simulink model "simula_RST_LPV"  (R2017a)
settings: Solver=VariableStepAuto  StartTime=0.0  StopTime=tsim  RelTol=1e-3
values from neighbouring files (symbols this model uses):
  Asim = double(A_LPV)    [Principal_LPV_RST.m]
  Bsim = double([zeros(1,d) B_LPV])    [Principal_LPV_RST.m]
  Rsim = double(R_LPV)    [Principal_LPV_RST.m]
  Ssim = double(S_LPV)    [Principal_LPV_RST.m]
  Ts = 0.05    [Principal_LPV_RST.m]
  Tsim = double(T_LPV)    [Principal_LPV_RST.m]
settings Model: Creator=FABRICIO  LastModifiedBy=FABRICIO

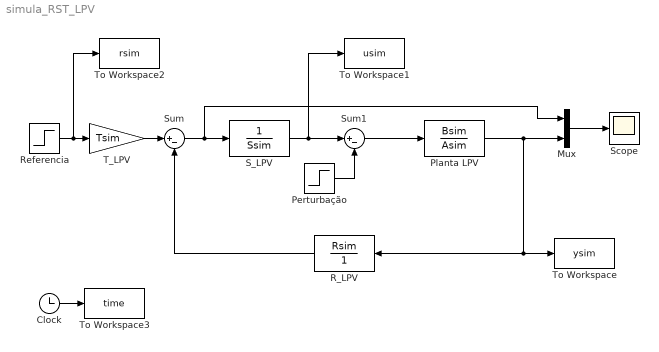
== system simula_RST_LPV ==
  Clock : Clock
  Mux : Mux  Inputs=2
  Perturbação : Step  Time=5  After=0.1  SampleTime=0
  Planta LPV : DiscreteFilter  Numerator=Bsim  Denominator=Asim  SampleTime=Ts
  R_LPV : DiscreteFilter  Numerator=Rsim  Denominator=1  SampleTime=Ts
  Referencia : Step  SampleTime=0
  S_LPV : DiscreteFilter  Numerator=1  Denominator=Ssim  SampleTime=Ts
  Scope : Scope
  Sum : Sum  Inputs=|+-
  Sum1 : Sum  Inputs=|+-
  T_LPV : Gain  Gain=Tsim
  To Workspace : ToWorkspace  VariableName=ysim  SampleTime=Ts
  To Workspace1 : ToWorkspace  VariableName=usim  SampleTime=Ts
  To Workspace2 : ToWorkspace  VariableName=rsim  SampleTime=Ts
  To Workspace3 : ToWorkspace  VariableName=time  SampleTime=Ts
  wires:
  Sum/1 -> Mux/1, S_LPV/1
  R_LPV/1 -> Sum/2
  Referencia/1 -> To Workspace2/1, T_LPV/1
  Mux/1 -> Scope/1
  T_LPV/1 -> Sum/1
  Clock/1 -> To Workspace3/1
  S_LPV/1 -> Sum1/1, To Workspace1/1
  Perturbação/1 -> Sum1/2
  Planta LPV/1 -> Mux/2, To Workspace/1, R_LPV/1
  Sum1/1 -> Planta LPV/1
